simulink model "test1"  (R2018a)
settings: Solver=FixedStepAuto  StartTime=0.0  StopTime=100  FixedStep=step_size  RelTol=1e-3  EnableMultiTasking=on
values from neighbouring files (symbols this model uses):
  alpha1 = 0.995    [DPEFOD.m]
  alpha2 = 0.075    [DPEFOD.m]
  B_bar = [A_hat'*inv(C_hat)*b1_hat;A_hat'*inv(C_hat)*b2_hat;A_hat'*inv(C_hat)*b3_hat;A_hat'*inv(C_hat)*b4_hat]    [DPEFOD.m]
  K_bar = kron(eye(4),A_hat'*inv(C_hat)*A_hat+rho*eye(5))+L_bar    [DPEFOD.m]
  L_bar = kron(L,eye(5))    [DPEFOD.m]
  lambda_0 = zeros(20,1)    [DPEFOD.m]
  theta_0 = zeros(20,1)    [DPEFOD.m]
(part 5 of 5)

== system test1/Subsystem2/Dawei integrator12 ==
  In1 : Inport
  Constant : Constant  Value=x0
  Sum : Sum  Inputs=|++
  Transfer Fcn : TransferFcn  Denominator=[T 1]
  Transfer Fcn1 : TransferFcn  Numerator=num  Denominator=den
  Out1 : Outport
  wires:
  Transfer Fcn1/1 -> Transfer Fcn/1
  In1/1 -> Transfer Fcn1/1
  Sum/1 -> Out1/1
  Transfer Fcn/1 -> Sum/1
  Constant/1 -> Sum/2

== system test1/Subsystem2/Dawei integrator13 ==
  In1 : Inport
  Constant : Constant  Value=x0
  Sum : Sum  Inputs=|++
  Transfer Fcn : TransferFcn  Denominator=[T 1]
  Transfer Fcn1 : TransferFcn  Numerator=num  Denominator=den
  Out1 : Outport
  wires:
  Transfer Fcn1/1 -> Transfer Fcn/1
  In1/1 -> Transfer Fcn1/1
  Sum/1 -> Out1/1
  Transfer Fcn/1 -> Sum/1
  Constant/1 -> Sum/2

== system test1/Subsystem2/Dawei integrator14 ==
  In1 : Inport
  Constant : Constant  Value=x0
  Sum : Sum  Inputs=|++
  Transfer Fcn : TransferFcn  Denominator=[T 1]
  Transfer Fcn1 : TransferFcn  Numerator=num  Denominator=den
  Out1 : Outport
  wires:
  Transfer Fcn1/1 -> Transfer Fcn/1
  In1/1 -> Transfer Fcn1/1
  Sum/1 -> Out1/1
  Transfer Fcn/1 -> Sum/1
  Constant/1 -> Sum/2

== system test1/Subsystem2/Dawei integrator15 ==
  In1 : Inport
  Constant : Constant  Value=x0
  Sum : Sum  Inputs=|++
  Transfer Fcn : TransferFcn  Denominator=[T 1]
  Transfer Fcn1 : TransferFcn  Numerator=num  Denominator=den
  Out1 : Outport
  wires:
  Transfer Fcn1/1 -> Transfer Fcn/1
  In1/1 -> Transfer Fcn1/1
  Sum/1 -> Out1/1
  Transfer Fcn/1 -> Sum/1
  Constant/1 -> Sum/2

== system test1/Subsystem2/Dawei integrator16 ==
  In1 : Inport
  Constant : Constant  Value=x0
  Sum : Sum  Inputs=|++
  Transfer Fcn : TransferFcn  Denominator=[T 1]
  Transfer Fcn1 : TransferFcn  Numerator=num  Denominator=den
  Out1 : Outport
  wires:
  Transfer Fcn1/1 -> Transfer Fcn/1
  In1/1 -> Transfer Fcn1/1
  Sum/1 -> Out1/1
  Transfer Fcn/1 -> Sum/1
  Constant/1 -> Sum/2

== system test1/Subsystem2/Dawei integrator17 ==
  In1 : Inport
  Constant : Constant  Value=x0
  Sum : Sum  Inputs=|++
  Transfer Fcn : TransferFcn  Denominator=[T 1]
  Transfer Fcn1 : TransferFcn  Numerator=num  Denominator=den
  Out1 : Outport
  wires:
  Transfer Fcn1/1 -> Transfer Fcn/1
  In1/1 -> Transfer Fcn1/1
  Sum/1 -> Out1/1
  Transfer Fcn/1 -> Sum/1
  Constant/1 -> Sum/2

== system test1/Subsystem2/Dawei integrator18 ==
  In1 : Inport
  Constant : Constant  Value=x0
  Sum : Sum  Inputs=|++
  Transfer Fcn : TransferFcn  Denominator=[T 1]
  Transfer Fcn1 : TransferFcn  Numerator=num  Denominator=den
  Out1 : Outport
  wires:
  Transfer Fcn1/1 -> Transfer Fcn/1
  In1/1 -> Transfer Fcn1/1
  Sum/1 -> Out1/1
  Transfer Fcn/1 -> Sum/1
  Constant/1 -> Sum/2

== system test1/Subsystem2/Dawei integrator19 ==
  In1 : Inport
  Constant : Constant  Value=x0
  Sum : Sum  Inputs=|++
  Transfer Fcn : TransferFcn  Denominator=[T 1]
  Transfer Fcn1 : TransferFcn  Numerator=num  Denominator=den
  Out1 : Outport
  wires:
  Transfer Fcn1/1 -> Transfer Fcn/1
  In1/1 -> Transfer Fcn1/1
  Sum/1 -> Out1/1
  Transfer Fcn/1 -> Sum/1
  Constant/1 -> Sum/2

== system test1/Subsystem2/Dawei integrator2 ==
  In1 : Inport
  Constant : Constant  Value=x0
  Sum : Sum  Inputs=|++
  Transfer Fcn : TransferFcn  Denominator=[T 1]
  Transfer Fcn1 : TransferFcn  Numerator=num  Denominator=den
  Out1 : Outport
  wires:
  Transfer Fcn1/1 -> Transfer Fcn/1
  In1/1 -> Transfer Fcn1/1
  Sum/1 -> Out1/1
  Transfer Fcn/1 -> Sum/1
  Constant/1 -> Sum/2

== system test1/Subsystem2/Dawei integrator20 ==
  In1 : Inport
  Constant : Constant  Value=x0
  Sum : Sum  Inputs=|++
  Transfer Fcn : TransferFcn  Denominator=[T 1]
  Transfer Fcn1 : TransferFcn  Numerator=num  Denominator=den
  Out1 : Outport
  wires:
  Transfer Fcn1/1 -> Transfer Fcn/1
  In1/1 -> Transfer Fcn1/1
  Sum/1 -> Out1/1
  Transfer Fcn/1 -> Sum/1
  Constant/1 -> Sum/2

== system test1/Subsystem2/Dawei integrator3 ==
  In1 : Inport
  Constant : Constant  Value=x0
  Sum : Sum  Inputs=|++
  Transfer Fcn : TransferFcn  Denominator=[T 1]
  Transfer Fcn1 : TransferFcn  Numerator=num  Denominator=den
  Out1 : Outport
  wires:
  Transfer Fcn1/1 -> Transfer Fcn/1
  In1/1 -> Transfer Fcn1/1
  Sum/1 -> Out1/1
  Transfer Fcn/1 -> Sum/1
  Constant/1 -> Sum/2

== system test1/Subsystem2/Dawei integrator4 ==
  In1 : Inport
  Constant : Constant  Value=x0
  Sum : Sum  Inputs=|++
  Transfer Fcn : TransferFcn  Denominator=[T 1]
  Transfer Fcn1 : TransferFcn  Numerator=num  Denominator=den
  Out1 : Outport
  wires:
  Transfer Fcn1/1 -> Transfer Fcn/1
  In1/1 -> Transfer Fcn1/1
  Sum/1 -> Out1/1
  Transfer Fcn/1 -> Sum/1
  Constant/1 -> Sum/2

== system test1/Subsystem2/Dawei integrator5 ==
  In1 : Inport
  Constant : Constant  Value=x0
  Sum : Sum  Inputs=|++
  Transfer Fcn : TransferFcn  Denominator=[T 1]
  Transfer Fcn1 : TransferFcn  Numerator=num  Denominator=den
  Out1 : Outport
  wires:
  Transfer Fcn1/1 -> Transfer Fcn/1
  In1/1 -> Transfer Fcn1/1
  Sum/1 -> Out1/1
  Transfer Fcn/1 -> Sum/1
  Constant/1 -> Sum/2

== system test1/Subsystem2/Dawei integrator6 ==
  In1 : Inport
  Constant : Constant  Value=x0
  Sum : Sum  Inputs=|++
  Transfer Fcn : TransferFcn  Denominator=[T 1]
  Transfer Fcn1 : TransferFcn  Numerator=num  Denominator=den
  Out1 : Outport
  wires:
  Transfer Fcn1/1 -> Transfer Fcn/1
  In1/1 -> Transfer Fcn1/1
  Sum/1 -> Out1/1
  Transfer Fcn/1 -> Sum/1
  Constant/1 -> Sum/2

== system test1/Subsystem2/Dawei integrator7 ==
  In1 : Inport
  Constant : Constant  Value=x0
  Sum : Sum  Inputs=|++
  Transfer Fcn : TransferFcn  Denominator=[T 1]
  Transfer Fcn1 : TransferFcn  Numerator=num  Denominator=den
  Out1 : Outport
  wires:
  Transfer Fcn1/1 -> Transfer Fcn/1
  In1/1 -> Transfer Fcn1/1
  Sum/1 -> Out1/1
  Transfer Fcn/1 -> Sum/1
  Constant/1 -> Sum/2

== system test1/Subsystem2/Dawei integrator8 ==
  In1 : Inport
  Constant : Constant  Value=x0
  Sum : Sum  Inputs=|++
  Transfer Fcn : TransferFcn  Denominator=[T 1]
  Transfer Fcn1 : TransferFcn  Numerator=num  Denominator=den
  Out1 : Outport
  wires:
  Transfer Fcn1/1 -> Transfer Fcn/1
  In1/1 -> Transfer Fcn1/1
  Sum/1 -> Out1/1
  Transfer Fcn/1 -> Sum/1
  Constant/1 -> Sum/2

== system test1/Subsystem2/Dawei integrator9 ==
  In1 : Inport
  Constant : Constant  Value=x0
  Sum : Sum  Inputs=|++
  Transfer Fcn : TransferFcn  Denominator=[T 1]
  Transfer Fcn1 : TransferFcn  Numerator=num  Denominator=den
  Out1 : Outport
  wires:
  Transfer Fcn1/1 -> Transfer Fcn/1
  In1/1 -> Transfer Fcn1/1
  Sum/1 -> Out1/1
  Transfer Fcn/1 -> Sum/1
  Constant/1 -> Sum/2

== system test1/Subsystem3/Dawei integrator1 ==
  In1 : Inport
  Constant : Constant  Value=x0
  Sum : Sum  Inputs=|++
  Transfer Fcn : TransferFcn  Denominator=[T 1]
  Transfer Fcn1 : TransferFcn  Numerator=num  Denominator=den
  Out1 : Outport
  wires:
  Transfer Fcn1/1 -> Transfer Fcn/1
  In1/1 -> Transfer Fcn1/1
  Sum/1 -> Out1/1
  Transfer Fcn/1 -> Sum/1
  Constant/1 -> Sum/2

== system test1/Subsystem3/Dawei integrator10 ==
  In1 : Inport
  Constant : Constant  Value=x0
  Sum : Sum  Inputs=|++
  Transfer Fcn : TransferFcn  Denominator=[T 1]
  Transfer Fcn1 : TransferFcn  Numerator=num  Denominator=den
  Out1 : Outport
  wires:
  Transfer Fcn1/1 -> Transfer Fcn/1
  In1/1 -> Transfer Fcn1/1
  Sum/1 -> Out1/1
  Transfer Fcn/1 -> Sum/1
  Constant/1 -> Sum/2

== system test1/Subsystem3/Dawei integrator11 ==
  In1 : Inport
  Constant : Constant  Value=x0
  Sum : Sum  Inputs=|++
  Transfer Fcn : TransferFcn  Denominator=[T 1]
  Transfer Fcn1 : TransferFcn  Numerator=num  Denominator=den
  Out1 : Outport
  wires:
  Transfer Fcn1/1 -> Transfer Fcn/1
  In1/1 -> Transfer Fcn1/1
  Sum/1 -> Out1/1
  Transfer Fcn/1 -> Sum/1
  Constant/1 -> Sum/2

== system test1/Subsystem3/Dawei integrator12 ==
  In1 : Inport
  Constant : Constant  Value=x0
  Sum : Sum  Inputs=|++
  Transfer Fcn : TransferFcn  Denominator=[T 1]
  Transfer Fcn1 : TransferFcn  Numerator=num  Denominator=den
  Out1 : Outport
  wires:
  Transfer Fcn1/1 -> Transfer Fcn/1
  In1/1 -> Transfer Fcn1/1
  Sum/1 -> Out1/1
  Transfer Fcn/1 -> Sum/1
  Constant/1 -> Sum/2

== system test1/Subsystem3/Dawei integrator13 ==
  In1 : Inport
  Constant : Constant  Value=x0
  Sum : Sum  Inputs=|++
  Transfer Fcn : TransferFcn  Denominator=[T 1]
  Transfer Fcn1 : TransferFcn  Numerator=num  Denominator=den
  Out1 : Outport
  wires:
  Transfer Fcn1/1 -> Transfer Fcn/1
  In1/1 -> Transfer Fcn1/1
  Sum/1 -> Out1/1
  Transfer Fcn/1 -> Sum/1
  Constant/1 -> Sum/2

== system test1/Subsystem3/Dawei integrator14 ==
  In1 : Inport
  Constant : Constant  Value=x0
  Sum : Sum  Inputs=|++
  Transfer Fcn : TransferFcn  Denominator=[T 1]
  Transfer Fcn1 : TransferFcn  Numerator=num  Denominator=den
  Out1 : Outport
  wires:
  Transfer Fcn1/1 -> Transfer Fcn/1
  In1/1 -> Transfer Fcn1/1
  Sum/1 -> Out1/1
  Transfer Fcn/1 -> Sum/1
  Constant/1 -> Sum/2

== system test1/Subsystem3/Dawei integrator15 ==
  In1 : Inport
  Constant : Constant  Value=x0
  Sum : Sum  Inputs=|++
  Transfer Fcn : TransferFcn  Denominator=[T 1]
  Transfer Fcn1 : TransferFcn  Numerator=num  Denominator=den
  Out1 : Outport
  wires:
  Transfer Fcn1/1 -> Transfer Fcn/1
  In1/1 -> Transfer Fcn1/1
  Sum/1 -> Out1/1
  Transfer Fcn/1 -> Sum/1
  Constant/1 -> Sum/2

== system test1/Subsystem3/Dawei integrator16 ==
  In1 : Inport
  Constant : Constant  Value=x0
  Sum : Sum  Inputs=|++
  Transfer Fcn : TransferFcn  Denominator=[T 1]
  Transfer Fcn1 : TransferFcn  Numerator=num  Denominator=den
  Out1 : Outport
  wires:
  Transfer Fcn1/1 -> Transfer Fcn/1
  In1/1 -> Transfer Fcn1/1
  Sum/1 -> Out1/1
  Transfer Fcn/1 -> Sum/1
  Constant/1 -> Sum/2

== system test1/Subsystem3/Dawei integrator17 ==
  In1 : Inport
  Constant : Constant  Value=x0
  Sum : Sum  Inputs=|++
  Transfer Fcn : TransferFcn  Denominator=[T 1]
  Transfer Fcn1 : TransferFcn  Numerator=num  Denominator=den
  Out1 : Outport
  wires:
  Transfer Fcn1/1 -> Transfer Fcn/1
  In1/1 -> Transfer Fcn1/1
  Sum/1 -> Out1/1
  Transfer Fcn/1 -> Sum/1
  Constant/1 -> Sum/2

== system test1/Subsystem3/Dawei integrator18 ==
  In1 : Inport
  Constant : Constant  Value=x0
  Sum : Sum  Inputs=|++
  Transfer Fcn : TransferFcn  Denominator=[T 1]
  Transfer Fcn1 : TransferFcn  Numerator=num  Denominator=den
  Out1 : Outport
  wires:
  Transfer Fcn1/1 -> Transfer Fcn/1
  In1/1 -> Transfer Fcn1/1
  Sum/1 -> Out1/1
  Transfer Fcn/1 -> Sum/1
  Constant/1 -> Sum/2

== system test1/Subsystem3/Dawei integrator19 ==
  In1 : Inport
  Constant : Constant  Value=x0
  Sum : Sum  Inputs=|++
  Transfer Fcn : TransferFcn  Denominator=[T 1]
  Transfer Fcn1 : TransferFcn  Numerator=num  Denominator=den
  Out1 : Outport
  wires:
  Transfer Fcn1/1 -> Transfer Fcn/1
  In1/1 -> Transfer Fcn1/1
  Sum/1 -> Out1/1
  Transfer Fcn/1 -> Sum/1
  Constant/1 -> Sum/2

== system test1/Subsystem3/Dawei integrator2 ==
  In1 : Inport
  Constant : Constant  Value=x0
  Sum : Sum  Inputs=|++
  Transfer Fcn : TransferFcn  Denominator=[T 1]
  Transfer Fcn1 : TransferFcn  Numerator=num  Denominator=den
  Out1 : Outport
  wires:
  Transfer Fcn1/1 -> Transfer Fcn/1
  In1/1 -> Transfer Fcn1/1
  Sum/1 -> Out1/1
  Transfer Fcn/1 -> Sum/1
  Constant/1 -> Sum/2

== system test1/Subsystem3/Dawei integrator20 ==
  In1 : Inport
  Constant : Constant  Value=x0
  Sum : Sum  Inputs=|++
  Transfer Fcn : TransferFcn  Denominator=[T 1]
  Transfer Fcn1 : TransferFcn  Numerator=num  Denominator=den
  Out1 : Outport
  wires:
  Transfer Fcn1/1 -> Transfer Fcn/1
  In1/1 -> Transfer Fcn1/1
  Sum/1 -> Out1/1
  Transfer Fcn/1 -> Sum/1
  Constant/1 -> Sum/2

== system test1/Subsystem3/Dawei integrator3 ==
  In1 : Inport
  Constant : Constant  Value=x0
  Sum : Sum  Inputs=|++
  Transfer Fcn : TransferFcn  Denominator=[T 1]
  Transfer Fcn1 : TransferFcn  Numerator=num  Denominator=den
  Out1 : Outport
  wires:
  Transfer Fcn1/1 -> Transfer Fcn/1
  In1/1 -> Transfer Fcn1/1
  Sum/1 -> Out1/1
  Transfer Fcn/1 -> Sum/1
  Constant/1 -> Sum/2

== system test1/Subsystem3/Dawei integrator4 ==
  In1 : Inport
  Constant : Constant  Value=x0
  Sum : Sum  Inputs=|++
  Transfer Fcn : TransferFcn  Denominator=[T 1]
  Transfer Fcn1 : TransferFcn  Numerator=num  Denominator=den
  Out1 : Outport
  wires:
  Transfer Fcn1/1 -> Transfer Fcn/1
  In1/1 -> Transfer Fcn1/1
  Sum/1 -> Out1/1
  Transfer Fcn/1 -> Sum/1
  Constant/1 -> Sum/2

== system test1/Subsystem3/Dawei integrator5 ==
  In1 : Inport
  Constant : Constant  Value=x0
  Sum : Sum  Inputs=|++
  Transfer Fcn : TransferFcn  Denominator=[T 1]
  Transfer Fcn1 : TransferFcn  Numerator=num  Denominator=den
  Out1 : Outport
  wires:
  Transfer Fcn1/1 -> Transfer Fcn/1
  In1/1 -> Transfer Fcn1/1
  Sum/1 -> Out1/1
  Transfer Fcn/1 -> Sum/1
  Constant/1 -> Sum/2

== system test1/Subsystem3/Dawei integrator6 ==
  In1 : Inport
  Constant : Constant  Value=x0
  Sum : Sum  Inputs=|++
  Transfer Fcn : TransferFcn  Denominator=[T 1]
  Transfer Fcn1 : TransferFcn  Numerator=num  Denominator=den
  Out1 : Outport
  wires:
  Transfer Fcn1/1 -> Transfer Fcn/1
  In1/1 -> Transfer Fcn1/1
  Sum/1 -> Out1/1
  Transfer Fcn/1 -> Sum/1
  Constant/1 -> Sum/2

== system test1/Subsystem3/Dawei integrator7 ==
  In1 : Inport
  Constant : Constant  Value=x0
  Sum : Sum  Inputs=|++
  Transfer Fcn : TransferFcn  Denominator=[T 1]
  Transfer Fcn1 : TransferFcn  Numerator=num  Denominator=den
  Out1 : Outport
  wires:
  Transfer Fcn1/1 -> Transfer Fcn/1
  In1/1 -> Transfer Fcn1/1
  Sum/1 -> Out1/1
  Transfer Fcn/1 -> Sum/1
  Constant/1 -> Sum/2

== system test1/Subsystem3/Dawei integrator8 ==
  In1 : Inport
  Constant : Constant  Value=x0
  Sum : Sum  Inputs=|++
  Transfer Fcn : TransferFcn  Denominator=[T 1]
  Transfer Fcn1 : TransferFcn  Numerator=num  Denominator=den
  Out1 : Outport
  wires:
  Transfer Fcn1/1 -> Transfer Fcn/1
  In1/1 -> Transfer Fcn1/1
  Sum/1 -> Out1/1
  Transfer Fcn/1 -> Sum/1
  Constant/1 -> Sum/2

== system test1/Subsystem3/Dawei integrator9 ==
  In1 : Inport
  Constant : Constant  Value=x0
  Sum : Sum  Inputs=|++
  Transfer Fcn : TransferFcn  Denominator=[T 1]
  Transfer Fcn1 : TransferFcn  Numerator=num  Denominator=den
  Out1 : Outport
  wires:
  Transfer Fcn1/1 -> Transfer Fcn/1
  In1/1 -> Transfer Fcn1/1
  Sum/1 -> Out1/1
  Transfer Fcn/1 -> Sum/1
  Constant/1 -> Sum/2
